simulink library "MeldasLibrary"  (R2016b)
settings: Solver=VariableStepAuto  StartTime=0.0  StopTime=10.0  RelTol=1e-3
libraries: simulink x2
settings Model: Creator=mulusoy  LastModifiedBy=mulusoy
settings DebuggingCC: SFUnconditionalPathOutOfParentDiag=warning  SFUnreachableStateOrJunctionDiag=warning  SFDanglingTransitionDiag=warning
settings CodeAppCC: CustomSymbolStrSimulinkFcn=$N
settings ConfigComp: CovMetricSettings=dswe

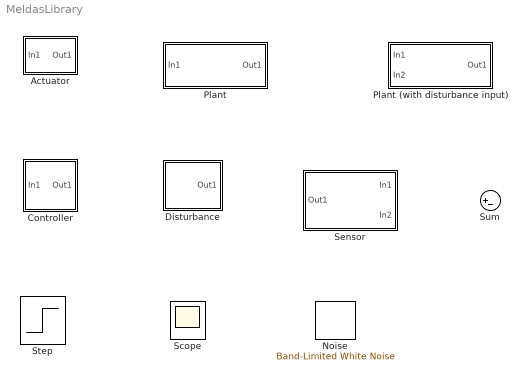
== system MeldasLibrary ==
  Actuator : Subsystem
      mask Display: image('.\Mask icons\Foot on pedal.png');
  Controller : Subsystem
      mask Display: image('.\Mask icons\Brain.jpg');
  Disturbance : Subsystem
      mask Display: image('.\Mask icons\Hill.jpg');
  Noise : simulink/Sources/Band-Limited White Noise  Cov=[0.01]  Ts=0.1  seed=[23341]
  Plant : Subsystem  Variant=on  mask{vehicleType=Car}
      mask prompts: vehicleType "Select Vehicle Type"
      mask TypeOptions vehicleType: Car | Sports car | Truck
      mask Callback vehicleType:
      | % Get the selected vehicle type
      | vehicleTypeStr = get_param(gcbh, 'vehicleType');
      | 
      | % Set the active variant
      | if strcmpi(vehicleTypeStr, 'car')
      |     evalin('base','vehicleType = 1;');
      | elseif strcmpi(vehicleTypeStr, 'sports car')
      |     evalin('base','vehicleType = 2;');
      | else
      |     evalin('base','vehicleType = 3;');
      | end
      mask Display:
      | % Update the icon based on the value of vehicleType
      | if vehicleType == 1
      |    image('.\Mask icons\Car.jpg');
      | elseif vehicleType == 2
      |    image('.\Mask icons\Sports car.jpg');
      | else
      |    image('.\Mask icons\Truck.jpg');
      | end
  Plant (with disturbance input) : Subsystem  Variant=on  mask{vehicleType=Car}
      mask prompts: vehicleType "Select Vehicle Type"
      mask TypeOptions vehicleType: Car | Sports car | Truck
      mask Callback vehicleType:
      | % Get the selected vehicle type
      | vehicleTypeStr = get_param(gcbh, 'vehicleType');
      | 
      | % Set the active variant
      | if strcmpi(vehicleTypeStr, 'car')
      |     evalin('base','vehicleType = 1;');
      | elseif strcmpi(vehicleTypeStr, 'sports car')
      |     evalin('base','vehicleType = 2;');
      | else
      |     evalin('base','vehicleType = 3;');
      | end
      mask Display:
      | % Update the icon based on the value of vehicleType
      | if vehicleType == 1
      |    image('.\Mask icons\Car.jpg');
      | elseif vehicleType == 2
      |    image('.\Mask icons\Sports car.jpg');
      | else
      |    image('.\Mask icons\Truck.jpg');
      | end
  Scope : Scope
  Sensor : Subsystem
      mask Display: image('.\Mask icons\Monitoring speed.jpg');
  Step : Step  After=20  SampleTime=0
  Sum : Sum  Inputs=|+-

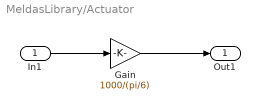
== system MeldasLibrary/Actuator ==
  In1 : Inport
  Gain : Gain  Gain=1000/(pi/6)
  Out1 : Outport
  wires:
  In1/1 -> Gain/1
  Gain/1 -> Out1/1

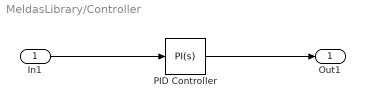
== system MeldasLibrary/Controller ==
  In1 : Inport
  PID Controller : simulink/Continuous/PID Controller  Controller=PI  TimeDomain=Continuous-time  SampleTime=-1  IntegratorMethod=Forward Euler  FilterMethod=Forward Euler  Form=Parallel  UseFilter=on  ControllerParametersSource=internal  P=0.111850088536406  I=0.00559250442682028  D=0  N=1.26652824631123  InitialConditionSource=internal  InitialConditionForIntegrator=0  InitialConditionForFilter=0  ExternalReset=none  LimitOutput=off  UpperSaturationLimit=12  LowerSaturationLimit=-12  LinearizeAsGain=on  AntiWindupMode=none  Kb=1  TrackingMode=off  Kt=1  PParamMin=[]  PParamMax=[]  IParamMin=[]  IParamMax=[]  DParamMin=[]  DParamMax=[]  NParamMin=[]  NParamMax=[]  KbParamMin=[]  KbParamMax=[]  KtParamMin=[]  KtParamMax=[]  POutMin=[]  POutMax=[]  IOutMin=[]  IOutMax=[]  DOutMin=[]  DOutMax=[]  NOutMin=[]  NOutMax=[]  KbOutMin=[]  KbOutMax=[]  KtOutMin=[]  KtOutMax=[]  IntegratorOutMin=[]  IntegratorOutMax=[]  FilterOutMin=[]  FilterOutMax=[]  SumOutMin=[]  SumOutMax=[]  SumI1OutMin=[]  SumI1OutMax=[]  SumI2OutMin=[]  SumI2OutMax=[]  SumI3OutMin=[]  SumI3OutMax=[]  SumDOutMin=[]  SumDOutMax=[]  SaturationOutMin=[]  SaturationOutMax=[]  IntegratorContinuousStateAttributes=''  IntegratorStateMustResolveToSignalObject=off  IntegratorRTWStateStorageClass=Auto  FilterContinuousStateAttributes=''  FilterStateMustResolveToSignalObject=off  FilterRTWStateStorageClass=Auto  DifferentiatorICPrevScaledInput=0  DifferentiatorOutMin=[]  DifferentiatorOutMax=[]
  Out1 : Outport
  wires:
  PID Controller/1 -> Out1/1
  In1/1 -> PID Controller/1

== system MeldasLibrary/Disturbance ==
  Step : Step  Time=200  After=-1000*9.81*sin(pi/45)  SampleTime=0
  Out1 : Outport
  wires:
  Step/1 -> Out1/1

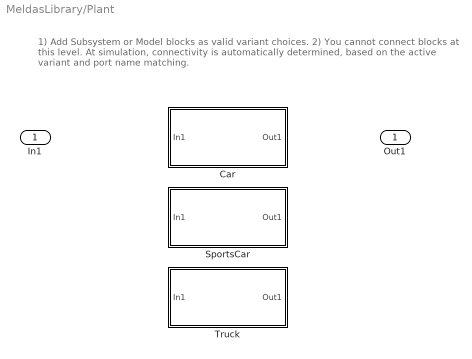
== system MeldasLibrary/Plant ==
  note: 1) Add Subsystem or Model blocks as valid variant choices.
      | 2) You cannot connect blocks at this level. At simulation, connectivity is automatically
      | determined, based on the active variant and port name matching.
  In1 : Inport
  Car : Subsystem  VariantControl=Car
      mask Display: image('.\Mask icons\Car.jpg');
  SportsCar : Subsystem  VariantControl=SportsCar
      mask Display: image('.\Mask icons\Sports car.jpg');
  Truck : Subsystem  VariantControl=Truck
      mask Display: image('.\Mask icons\Truck.jpg');
  Out1 : Outport

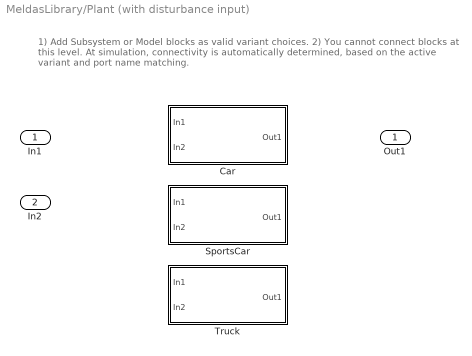
== system MeldasLibrary/Plant (with disturbance input) ==
  note: 1) Add Subsystem or Model blocks as valid variant choices.
      | 2) You cannot connect blocks at this level. At simulation, connectivity is automatically
      | determined, based on the active variant and port name matching.
  In1 : Inport
  In2 : Inport  Port=2
  Car : Subsystem  VariantControl=Car
      mask Display: image('.\Mask icons\Car.jpg');
  SportsCar : Subsystem  VariantControl=SportsCar
      mask Display: image('.\Mask icons\Sports car.jpg');
  Truck : Subsystem  VariantControl=Truck
      mask Display: image('.\Mask icons\Truck.jpg');
  Out1 : Outport

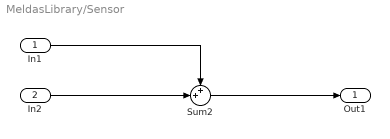
== system MeldasLibrary/Sensor ==
  In1 : Inport
  In2 : Inport  Port=2
  Sum2 : Sum  Inputs=++|
  Out1 : Outport
  wires:
  In1/1 -> Sum2/1
  In2/1 -> Sum2/2
  Sum2/1 -> Out1/1

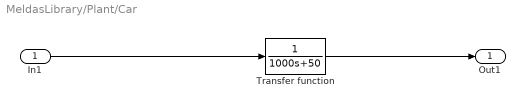
== system MeldasLibrary/Plant/Car ==
  "In1 " : Inport
  Transfer function : TransferFcn  Denominator=[1000 50]
  Out1 : Outport
  wires:
  "In1 "/1 -> Transfer function/1
  Transfer function/1 -> Out1/1

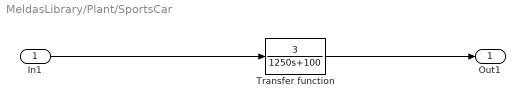
== system MeldasLibrary/Plant/SportsCar ==
  "In1 " : Inport
  Transfer function : TransferFcn  Numerator=[3]  Denominator=[1250 100]
  Out1 : Outport
  wires:
  Transfer function/1 -> Out1/1
  "In1 "/1 -> Transfer function/1

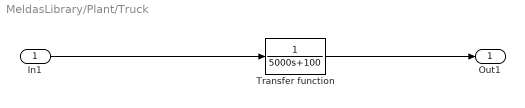
== system MeldasLibrary/Plant/Truck ==
  "In1 " : Inport
  Transfer function : TransferFcn  Denominator=[5000 100]
  Out1 : Outport
  wires:
  "In1 "/1 -> Transfer function/1
  Transfer function/1 -> Out1/1

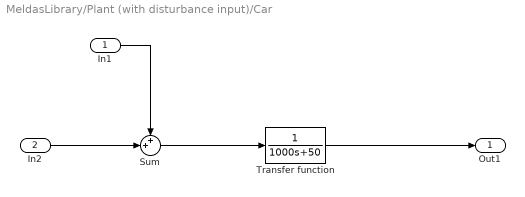
== system MeldasLibrary/Plant (with disturbance input)/Car ==
  In1 : Inport
  "In2 " : Inport  Port=2
  Sum : Sum  Inputs=++|
  Transfer function : TransferFcn  Denominator=[1000 50]
  Out1 : Outport
  wires:
  Transfer function/1 -> Out1/1
  "In2 "/1 -> Sum/2
  In1/1 -> Sum/1
  Sum/1 -> Transfer function/1

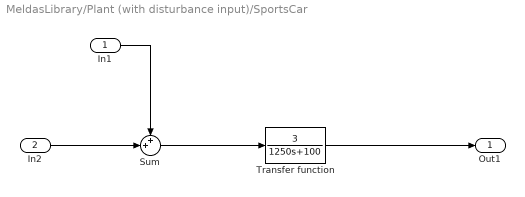
== system MeldasLibrary/Plant (with disturbance input)/SportsCar ==
  In1 : Inport
  "In2 " : Inport  Port=2
  Sum : Sum  Inputs=++|
  Transfer function : TransferFcn  Numerator=[3]  Denominator=[1250 100]
  Out1 : Outport
  wires:
  Sum/1 -> Transfer function/1
  In1/1 -> Sum/1
  "In2 "/1 -> Sum/2
  Transfer function/1 -> Out1/1

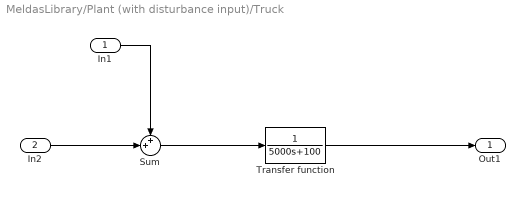
== system MeldasLibrary/Plant (with disturbance input)/Truck ==
  In1 : Inport
  "In2 " : Inport  Port=2
  Sum : Sum  Inputs=++|
  Transfer function : TransferFcn  Denominator=[5000 100]
  Out1 : Outport
  wires:
  Transfer function/1 -> Out1/1
  "In2 "/1 -> Sum/2
  In1/1 -> Sum/1
  Sum/1 -> Transfer function/1
